simulink model "UUV_FD"  (R2018a)
settings: Solver=FixedStepAuto  StartTime=0.0  StopTime=25  FixedStep=0.01  RelTol=1e-3  EnableMultiTasking=on
settings Model: Creator=Alireza  LastModifiedBy=7385281
settings DataIOCC: LimitDataPoints=on  SaveFormat=Array  SignalLoggingSaveFormat=ModelDataLogs
settings OptimizationCC: ExpressionDepthLimit=2147483647  LifeSpan=inf
settings DebuggingCC: UnderspecifiedInitializationDetection=Classic  MergeDetectMultiDrivingBlocksExec=none  SolverPrmCheckMsg=warning  FcnCallInpInsideContextMsg=warning  AllowSymbolicDim=off  StateNameClashWarn=warning  SFUnexpectedBacktrackingDiag=warning  SFNoUnconditionalDefaultTransitionDiag=warning  SFExecutionAtInitializationDiag=none
settings HardwareCC: ProdBitPerPointer=32  ProdBitPerSizeT=32  ProdBitPerPtrDiffT=32  ProdLargestAtomicFloat=None  ProdIntDivRoundTo=Undefined  ProdEndianess=Unspecified  ProdWordSize=32  ProdHWDeviceType=32-bit Generic
settings ModelReferenceCC: PropagateSignalLabelsOutOfModel=off
settings CodeAppCC: StateflowObjectComments=on
settings GRTTargetCC: TargetLangStandard=C89/C90 (ANSI)  GeneratePreprocessorConditionals=Disable all  CombineOutputUpdateFcns=off  GRTInterface=on
settings ConfigComp: CovMetricSettings=dw  CovHtmlReporting=on  CovSaveCumulativeToWorkspaceVar=on  CovSaveSingleToWorkspaceVar=on  CovExternalEMLEnable=off

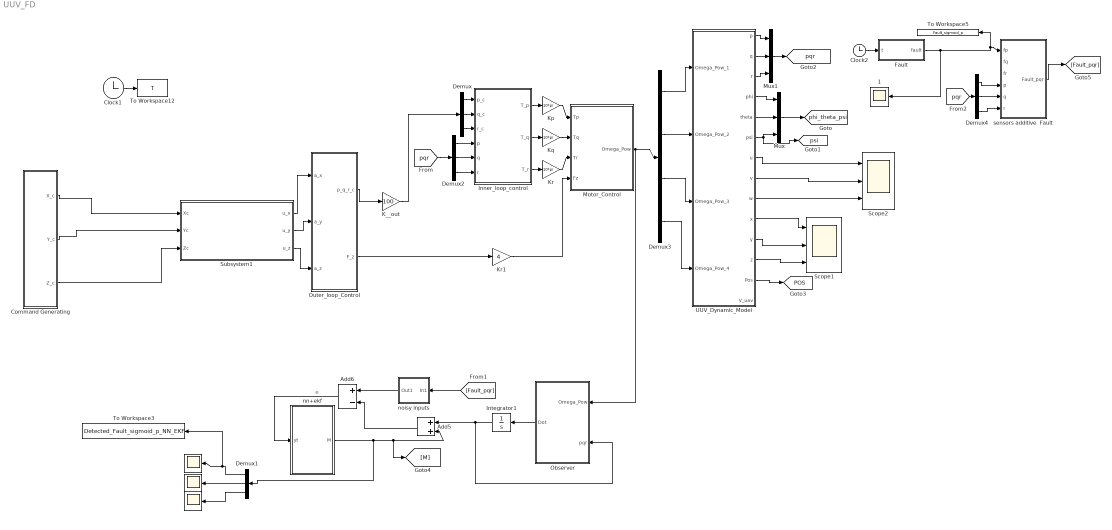
== system UUV_FD ==
  note: e
  "     " : Scope
  "      " : Scope
  "          " : Scope
  "     1" : Scope
  Add5 : Sum
  Add6 : Sum  Inputs=+-  OutDataTypeStr=Inherit: Same as accumulator
  Clock1 : Clock
  Clock2 : Clock
  Command Generating : Subsystem
  Demux{,1..2,4} (4 alike) : Demux  Outputs=3
  Demux3 : Demux
  Fault : MATLAB Function  TreatAsAtomicUnit=on
  Inner_loop_control : MATLAB Function  TreatAsAtomicUnit=on
  Integrator1 : Integrator  InitialCondition=[0.0001;0.0001;0.0001]
  K__out : Gain  Gain=100
  Kp : Gain  Gain=10*pi
  Kq : Gain  Gain=10*pi
  Kr : Gain  Gain=10*pi
  Kr1 : Gain  Gain=4
  Motor_Control : MATLAB Function  TreatAsAtomicUnit=on
  Mux : Mux  Inputs=3
  Mux1 : Mux  Inputs=3
  Observer : MATLAB Function  TreatAsAtomicUnit=on
  Outer_loop_Control : Subsystem
  Scope1 : Scope  NumInputPorts=3
  Scope2 : Scope  NumInputPorts=3
  Subsystem1 : Subsystem
  To Workspace12 : ToWorkspace  VariableName=T  SampleTime=-1
  To Workspace3 : ToWorkspace  VariableName=Detected_Fault_sigmoid_p_NN_EKF  SampleTime=-1
  To Workspace5 : ToWorkspace  VariableName=Fault_sigmoid_p  SampleTime=-1
  UUV_Dynamic_Model : Subsystem
  nn+ekf : Subsystem
  noisy inputs : Subsystem
  "sensors additive  Fault " : MATLAB Function  TreatAsAtomicUnit=on
  tag scope: POS=global, phi_theta_psi=global, pqr=global, psi=global
  wires:
  UUV_Dynamic_Model/4(phi) -> Mux/1
  UUV_Dynamic_Model/5(theta) -> Mux/2
  UUV_Dynamic_Model/6(psi) -> [psi], Mux/3
  Mux/1 -> [phi_theta_psi]
  Inner_loop_control/1(T_p) -> Kp/1
  Inner_loop_control/2(T_q) -> Kq/1
  Inner_loop_control/3(T_r) -> Kr/1
  UUV_Dynamic_Model/1(p) -> Mux1/1
  UUV_Dynamic_Model/2(q) -> Mux1/2
  UUV_Dynamic_Model/3(r) -> Mux1/3
  Mux1/1 -> [pqr]
  Demux2/1 -> Inner_loop_control/4(p)
  Demux2/2 -> Inner_loop_control/5(q)
  Demux2/3 -> Inner_loop_control/6(r)
  [pqr] -> Demux2/1
  K__out/1 -> Demux/1
  Demux/1 -> Inner_loop_control/1(p_c)
  Demux/2 -> Inner_loop_control/2(q_c)
  Demux/3 -> Inner_loop_control/3(r_c)
  UUV_Dynamic_Model/10(x) -> Scope1/1
  UUV_Dynamic_Model/11(y) -> Scope1/2
  UUV_Dynamic_Model/12(z) -> Scope1/3
  UUV_Dynamic_Model/7(u) -> Scope2/1
  UUV_Dynamic_Model/8(v) -> Scope2/2
  UUV_Dynamic_Model/9(w) -> Scope2/3
  UUV_Dynamic_Model/13(Pos) -> [POS]
  Motor_Control/1(Omega_Pow) -> Demux3/1, Observer/1(Omega_Pow)
  Demux3/1 -> UUV_Dynamic_Model/1(Omega_Pow_1)
  Demux3/3 -> UUV_Dynamic_Model/3(Omega_Pow_3)
  Demux3/4 -> UUV_Dynamic_Model/4(Omega_Pow_4)
  Kp/1 -> Motor_Control/1(Tp)
  Kq/1 -> Motor_Control/2(Tq)
  Kr/1 -> Motor_Control/3(Tr)
  Demux3/2 -> UUV_Dynamic_Model/2(Omega_Pow_2)
  Command Generating/1(X_c) -> Subsystem1/1(Xc)
  Command Generating/2(Y_c) -> Subsystem1/2(Yc)
  Command Generating/3(Z_c) -> Subsystem1/3(Zc)
  Clock1/1 -> To Workspace12/1
  Subsystem1/1(u_x) -> Outer_loop_Control/1(a_x)
  Subsystem1/2(u_y) -> Outer_loop_Control/2(a_y)
  Subsystem1/3(u_z) -> Outer_loop_Control/3(a_z)
  Outer_loop_Control/1(p_q_r_c) -> K__out/1
  Outer_loop_Control/2(F_z) -> Kr1/1
  Kr1/1 -> Motor_Control/4(Fz)
  "sensors additive  Fault "/1(Fault_pqr) -> [Fault_pqr]
  Fault/1(fault) -> To Workspace5/1, "sensors additive  Fault "/1(fp), "     1"/1
  Observer/1(Dot) -> Integrator1/1
  Integrator1/1 -> Add5/1, Observer/2(pqr)
  Add5/1 -> Add6/2
  Add6/1 -> nn+ekf/1(yt)
  nn+ekf/1(M) -> Add5/2, [M], Demux1/1
  Demux1/3 -> "          "/1
  Demux1/1 -> "     "/1, To Workspace3/1
  Demux1/2 -> "      "/1
  [Fault_pqr] -> noisy inputs/1(In1)
  noisy inputs/1(Out1) -> Add6/1
  [pqr] -> Demux4/1
  Demux4/3 -> "sensors additive  Fault "/6(r)
  Demux4/2 -> "sensors additive  Fault "/5(q)
  Demux4/1 -> "sensors additive  Fault "/4(p)
  Clock2/1 -> Fault/1(t)

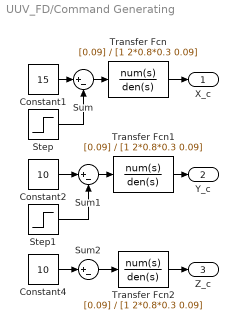
== system UUV_FD/Command Generating ==
  Constant1 : Constant  Value=15
  Constant2 : Constant  Value=10
  Constant4 : Constant  Value=10
  Step : Step  Time=30  After=15  SampleTime=0
  Step1 : Step  Time=15  After=10  SampleTime=0
  Sum : Sum  Inputs=|+-
  Sum1 : Sum  Inputs=|+-
  Sum2 : Sum  Inputs=|+-
  Transfer Fcn : TransferFcn  Numerator=[0.09]  Denominator=[1 2*0.8*0.3 0.09]
  Transfer Fcn1 : TransferFcn  Numerator=[0.09]  Denominator=[1 2*0.8*0.3 0.09]
  Transfer Fcn2 : TransferFcn  Numerator=[0.09]  Denominator=[1 2*0.8*0.3 0.09]
  X_c : Outport
  Y_c : Outport  Port=2
  Z_c : Outport  Port=3
  wires:
  Constant4/1 -> Sum2/1
  Transfer Fcn1/1 -> Y_c/1
  Transfer Fcn/1 -> X_c/1
  Constant2/1 -> Sum1/1
  Constant1/1 -> Sum/1
  Step/1 -> Sum/2
  Sum/1 -> Transfer Fcn/1
  Sum1/1 -> Transfer Fcn1/1
  Sum2/1 -> Transfer Fcn2/1
  Step1/1 -> Sum1/2
  Transfer Fcn2/1 -> Z_c/1

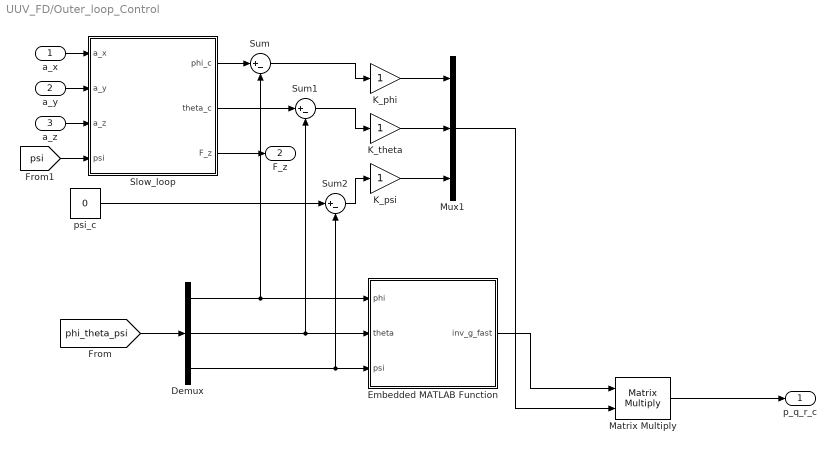
== system UUV_FD/Outer_loop_Control ==
  a_x : Inport
  a_y : Inport  Port=2
  a_z : Inport  Port=3
  Demux : Demux  Outputs=3
  Embedded MATLAB Function : MATLAB Function  TreatAsAtomicUnit=on
  K_phi : Gain
  K_psi : Gain
  K_theta : Gain
  Matrix Multiply : Product  Multiplication=Matrix(*)
  Mux1 : Mux  Inputs=3
  Slow_loop : MATLAB Function  TreatAsAtomicUnit=on
  Sum : Sum  Inputs=|+-
  Sum1 : Sum  Inputs=|+-
  Sum2 : Sum  Inputs=|+-
  psi_c : Constant  Value=0
  p_q_r_c : Outport
  F_z : Outport  Port=2
  wires:
  Sum1/1 -> K_theta/1
  Slow_loop/2(theta_c) -> Sum1/1
  Sum/1 -> K_phi/1
  Slow_loop/1(phi_c) -> Sum/1
  [phi_theta_psi] -> Demux/1
  Demux/1 -> Embedded MATLAB Function/1(phi), Sum/2
  Demux/2 -> Embedded MATLAB Function/2(theta), Sum1/2
  Demux/3 -> Embedded MATLAB Function/3(psi), Sum2/2
  psi_c/1 -> Sum2/1
  Sum2/1 -> K_psi/1
  [psi] -> Slow_loop/4(psi)
  K_phi/1 -> Mux1/1
  K_theta/1 -> Mux1/2
  K_psi/1 -> Mux1/3
  a_x/1 -> Slow_loop/1(a_x)
  a_y/1 -> Slow_loop/2(a_y)
  a_z/1 -> Slow_loop/3(a_z)
  Mux1/1 -> Matrix Multiply/2
  Slow_loop/3(F_z) -> F_z/1
  Embedded MATLAB Function/1(inv_g_fast) -> Matrix Multiply/1
  Matrix Multiply/1 -> p_q_r_c/1

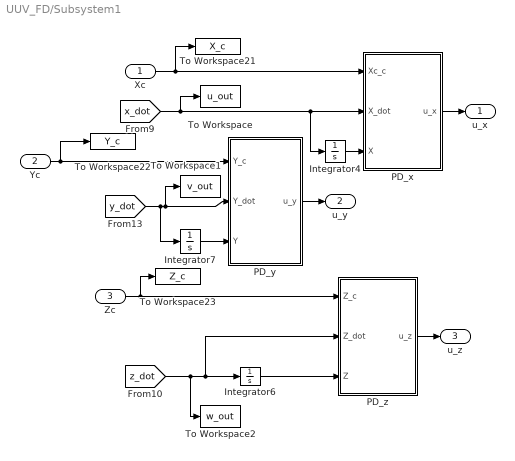
== system UUV_FD/Subsystem1 ==
  Xc : Inport
  Yc : Inport  Port=2
  Zc : Inport  Port=3
  Integrator4 : Integrator
  Integrator6 : Integrator
  Integrator7 : Integrator
  PD_x : Subsystem
  PD_y : Subsystem
  PD_z : Subsystem
  To Workspace : ToWorkspace  VariableName=u_out  SampleTime=-1
  To Workspace1 : ToWorkspace  VariableName=v_out  SampleTime=-1
  To Workspace2 : ToWorkspace  VariableName=w_out  SampleTime=-1
  To Workspace21 : ToWorkspace  VariableName=X_c  SampleTime=-1
  To Workspace22 : ToWorkspace  VariableName=Y_c  SampleTime=-1
  To Workspace23 : ToWorkspace  VariableName=Z_c  SampleTime=-1
  u_x : Outport
  u_y : Outport  Port=2
  u_z : Outport  Port=3
  wires:
  PD_z/1(u_z) -> u_z/1
  PD_y/1(u_y) -> u_y/1
  PD_x/1(u_x) -> u_x/1
  Zc/1 -> PD_z/1(Z_c), To Workspace23/1
  Yc/1 -> To Workspace22/1, PD_y/1(Y_c)
  Xc/1 -> PD_x/1(Xc_c), To Workspace21/1
  Integrator7/1 -> PD_y/3(Y)
  [x_dot] -> To Workspace/1, Integrator4/1, PD_x/2(X_dot)
  Integrator4/1 -> PD_x/3(X)
  [y_dot] -> PD_y/2(Y_dot), To Workspace1/1, Integrator7/1
  [z_dot] -> To Workspace2/1, Integrator6/1, PD_z/2(Z_dot)
  Integrator6/1 -> PD_z/3(Z)

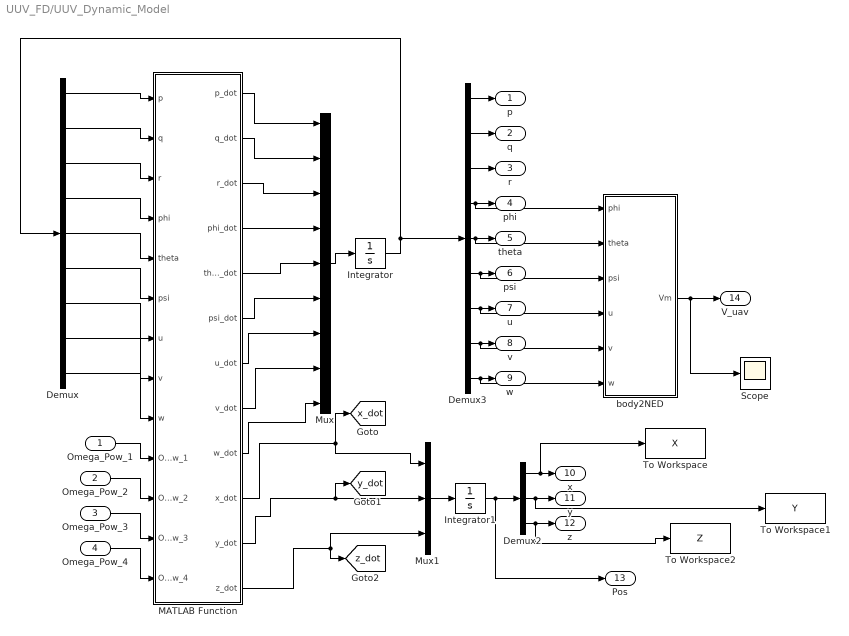
== system UUV_FD/UUV_Dynamic_Model ==
  Omega_Pow_1 : Inport
  Omega_Pow_2 : Inport  Port=2
  Omega_Pow_3 : Inport  Port=3
  Omega_Pow_4 : Inport  Port=4
  Demux : Demux  Outputs=9
  Demux2 : Demux  Outputs=3
  Demux3 : Demux  Outputs=9
  Integrator : Integrator  InitialCondition=[0.0001;0.0001;0.0001;0.00001;0.0001;0.0001;0.0001;0.0001;0.0001]
  Integrator1 : Integrator
  MATLAB Function : MATLAB Function  TreatAsAtomicUnit=on
  Mux : Mux  Inputs=9
  Mux1 : Mux  Inputs=3
  Scope : Scope
  To Workspace : ToWorkspace  VariableName=X  SampleTime=-1
  To Workspace1 : ToWorkspace  VariableName=Y  SampleTime=-1
  To Workspace2 : ToWorkspace  VariableName=Z  SampleTime=-1
  body2NED : MATLAB Function  TreatAsAtomicUnit=on
  p : Outport
  q : Outport  Port=2
  r : Outport  Port=3
  phi : Outport  Port=4
  theta : Outport  Port=5
  psi : Outport  Port=6
  u : Outport  Port=7
  v : Outport  Port=8
  w : Outport  Port=9
  x : Outport  Port=10
  y : Outport  Port=11
  z : Outport  Port=12
  Pos : Outport  Port=13
  V_uav : Outport  Port=14
  tag scope: x_dot=global, y_dot=global, z_dot=global
  wires:
  MATLAB Function/1(p_dot) -> Mux/1
  MATLAB Function/2(q_dot) -> Mux/2
  MATLAB Function/3(r_dot) -> Mux/3
  MATLAB Function/4(phi_dot) -> Mux/4
  MATLAB Function/5(theta_dot) -> Mux/5
  MATLAB Function/6(psi_dot) -> Mux/6
  MATLAB Function/7(u_dot) -> Mux/7
  MATLAB Function/8(v_dot) -> Mux/8
  MATLAB Function/9(w_dot) -> Mux/9
  Mux/1 -> Integrator/1
  Demux/1 -> MATLAB Function/1(p)
  Demux/2 -> MATLAB Function/2(q)
  Demux/3 -> MATLAB Function/3(r)
  Demux/4 -> MATLAB Function/4(phi)
  Demux/5 -> MATLAB Function/5(theta)
  Demux/6 -> MATLAB Function/6(psi)
  Demux/7 -> MATLAB Function/7(u)
  Demux/8 -> MATLAB Function/8(v)
  Demux/9 -> MATLAB Function/9(w)
  Integrator/1 -> Demux/1, Demux3/1
  MATLAB Function/10(x_dot) -> [x_dot], Mux1/1
  MATLAB Function/11(y_dot) -> Mux1/2, [y_dot]
  MATLAB Function/12(z_dot) -> [z_dot], Mux1/3
  Mux1/1 -> Integrator1/1
  Integrator1/1 -> Demux2/1, Pos/1
  Demux3/1 -> p/1
  Demux3/2 -> q/1
  Demux3/3 -> r/1
  Demux3/4 -> phi/1, body2NED/1(phi)
  Demux3/5 -> theta/1, body2NED/2(theta)
  Demux3/6 -> psi/1, body2NED/3(psi)
  Demux3/7 -> u/1, body2NED/4(u)
  Demux3/8 -> v/1, body2NED/5(v)
  Demux3/9 -> w/1, body2NED/6(w)
  Omega_Pow_1/1 -> MATLAB Function/10(Omega_Pow_1)
  Demux2/1 -> x/1, To Workspace/1
  Demux2/2 -> y/1, To Workspace1/1
  Omega_Pow_2/1 -> MATLAB Function/11(Omega_Pow_2)
  Demux2/3 -> z/1, To Workspace2/1
  Omega_Pow_3/1 -> MATLAB Function/12(Omega_Pow_3)
  Omega_Pow_4/1 -> MATLAB Function/13(Omega_Pow_4)
  body2NED/1(Vm) -> V_uav/1, Scope/1

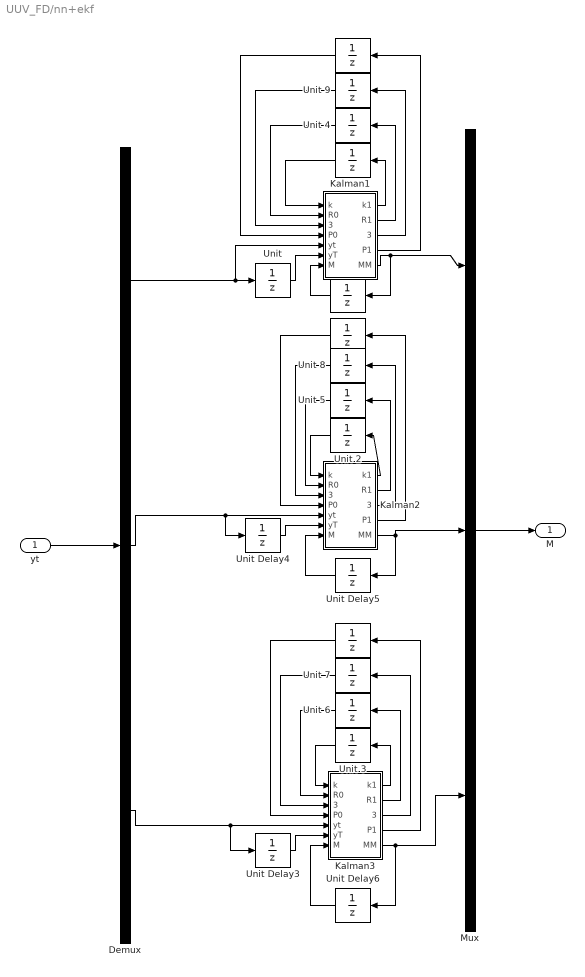
== system UUV_FD/nn+ekf ==
  yt : Inport
  " " : UnitDelay  InitialCondition=1  SampleTime=-1
  "  " : UnitDelay  InitialCondition=5*eye(3)  SampleTime=-1
  "   " : UnitDelay  InitialCondition=5*eye(3)  SampleTime=-1
  "      " : UnitDelay  InitialCondition=.01  SampleTime=-1
  "                " : UnitDelay  InitialCondition=10*eye(3)  SampleTime=-1
  Demux : Demux  Outputs=3
  Kalman1 : MATLAB Function  TreatAsAtomicUnit=on
  Kalman2 : MATLAB Function  TreatAsAtomicUnit=on
  Kalman3 : MATLAB Function  TreatAsAtomicUnit=on
  Mux : Mux  Inputs=3
  "Unit " : UnitDelay  SampleTime=-1
  Unit 2 : UnitDelay  InitialCondition=1  SampleTime=-1
  Unit 3 : UnitDelay  InitialCondition=1  SampleTime=-1
  Unit 4 : UnitDelay  InitialCondition=.00002  SampleTime=-1
  Unit 5 : UnitDelay  InitialCondition=.00002  SampleTime=-1
  Unit 6 : UnitDelay  InitialCondition=.00002  SampleTime=-1
  Unit 7 : UnitDelay  InitialCondition=[1;1;1]  SampleTime=-1
  Unit 8 : UnitDelay  InitialCondition=[1;.5;.5]  SampleTime=-1
  Unit 9 : UnitDelay  InitialCondition=[1;.5;.5]  SampleTime=-1
  Unit Delay3 : UnitDelay  SampleTime=-1
  Unit Delay4 : UnitDelay  SampleTime=-1
  Unit Delay5 : UnitDelay  InitialCondition=.01  SampleTime=-1
  Unit Delay6 : UnitDelay  InitialCondition=.01  SampleTime=-1
  M : Outport
  wires:
  "                "/1 -> Kalman3/4(P0)
  Kalman3/4(P1) -> "                "/1
  "   "/1 -> Kalman2/4(P0)
  Kalman2/4(P1) -> "   "/1
  Unit 8/1 -> Kalman2/3(teta0)
  Kalman2/3(teta1) -> Unit 8/1
  Unit 7/1 -> Kalman3/3(teta0)
  Kalman3/3(teta1) -> Unit 7/1
  Unit 6/1 -> Kalman3/2(R0)
  Kalman3/2(R1) -> Unit 6/1
  Unit 5/1 -> Kalman2/2(R0)
  Kalman2/2(R1) -> Unit 5/1
  Unit 3/1 -> Kalman3/1(k)
  Kalman3/1(k1) -> Unit 3/1
  Unit 2/1 -> Kalman2/1(k)
  Kalman2/1(k1) -> Unit 2/1
  Kalman3/5(MM) -> Unit Delay6/1, Mux/3
  Unit Delay5/1 -> Kalman2/7(M)
  Unit Delay4/1 -> Kalman2/6(yT)
  Unit Delay6/1 -> Kalman3/7(M)
  Unit Delay3/1 -> Kalman3/6(yT)
  Demux/2 -> Kalman2/5(yt), Unit Delay4/1
  Kalman2/5(MM) -> Unit Delay5/1, Mux/2
  Demux/3 -> Kalman3/5(yt), Unit Delay3/1
  Mux/1 -> M/1
  yt/1 -> Demux/1
  "  "/1 -> Kalman1/4(P0)
  Kalman1/4(P1) -> "  "/1
  Unit 9/1 -> Kalman1/3(teta0)
  Kalman1/3(teta1) -> Unit 9/1
  Unit 4/1 -> Kalman1/2(R0)
  Kalman1/2(R1) -> Unit 4/1
  " "/1 -> Kalman1/1(k)
  Kalman1/1(k1) -> " "/1
  "      "/1 -> Kalman1/7(M)
  "Unit "/1 -> Kalman1/6(yT)
  Demux/1 -> Kalman1/5(yt), "Unit "/1
  Kalman1/5(MM) -> "      "/1, Mux/1

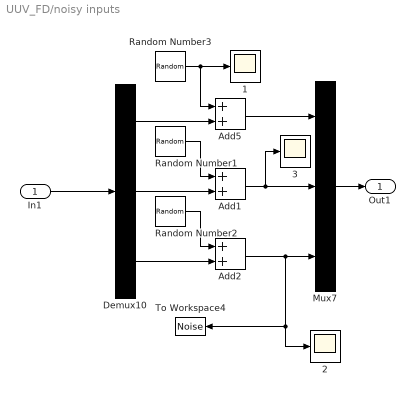
== system UUV_FD/noisy inputs ==
  In1 : Inport
  "     1" : Scope
  "     2" : Scope
  "     3" : Scope
  Add1 : Sum
  Add2 : Sum
  Add5 : Sum
  Demux10 : Demux  Outputs=3
  Mux7 : Mux  Inputs=3
  Random Number1 : RandomNumber  Variance=(1*pi/180)^2  Seed=18
  Random Number2 : RandomNumber  Variance=(1*pi/180)^2  Seed=40
  Random Number3 : RandomNumber  Variance=(1*pi/180)^2  Seed=68
  To Workspace4 : ToWorkspace  VariableName=Noise  SampleTime=-1
  Out1 : Outport
  wires:
  In1/1 -> Demux10/1
  Mux7/1 -> Out1/1
  Random Number3/1 -> Add5/1, "     1"/1
  Demux10/1 -> Add5/2
  Add5/1 -> Mux7/1
  Random Number1/1 -> Add1/1
  Demux10/2 -> Add1/2
  Add1/1 -> Mux7/2, "     3"/1
  Random Number2/1 -> Add2/1
  Demux10/3 -> Add2/2
  Add2/1 -> Mux7/3, "     2"/1, To Workspace4/1

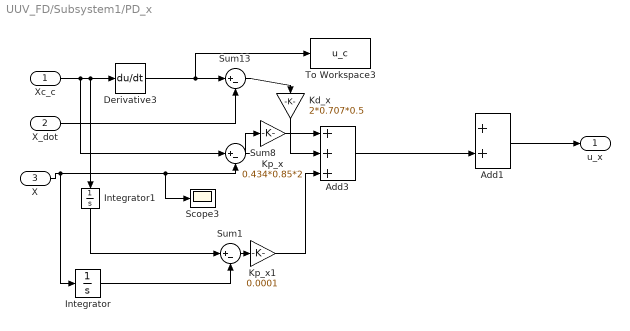
== system UUV_FD/Subsystem1/PD_x ==
  Xc_c : Inport
  X_dot : Inport  Port=2
  X : Inport  Port=3
  Add1 : Sum
  Add3 : Sum  Inputs=+++
  Derivative3 : Derivative
  Integrator : Integrator
  Integrator1 : Integrator
  Kd_x : Gain  Gain=2*0.707*0.5
  Kp_x : Gain  Gain=0.434*0.85*2
  Kp_x1 : Gain  Gain=0.0001
  Scope3 : Scope
  Sum1 : Sum  Inputs=|+-
  Sum13 : Sum  Inputs=|+-
  Sum8 : Sum  Inputs=|+-
  To Workspace3 : ToWorkspace  VariableName=u_c  SampleTime=-1
  u_x : Outport
  wires:
  Add3/1 -> Add1/2
  Add1/1 -> u_x/1
  Kp_x1/1 -> Add3/3
  Integrator1/1 -> Sum1/1
  Integrator/1 -> Sum1/2
  Sum1/1 -> Kp_x1/1
  X_dot/1 -> Sum13/2
  Xc_c/1 -> Integrator1/1, Derivative3/1, Sum8/1
  Kp_x/1 -> Add3/2
  Kd_x/1 -> Add3/1
  Sum13/1 -> Kd_x/1
  Derivative3/1 -> To Workspace3/1, Sum13/1
  X/1 -> Integrator/1, Sum8/2, Scope3/1
  Sum8/1 -> Kp_x/1

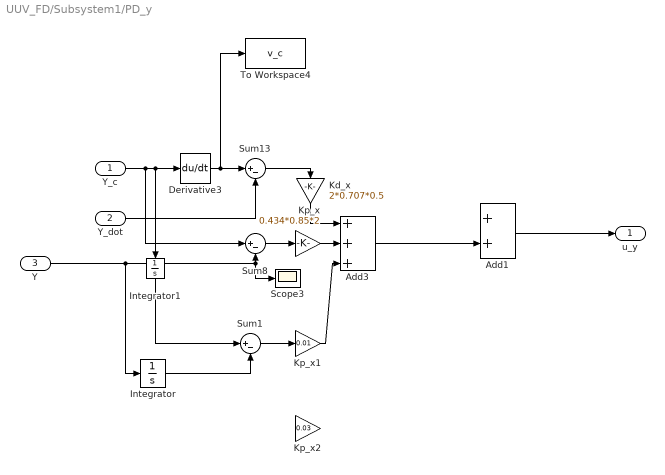
== system UUV_FD/Subsystem1/PD_y ==
  Y_c : Inport
  Y_dot : Inport  Port=2
  Y : Inport  Port=3
  Add1 : Sum
  Add3 : Sum  Inputs=+++
  Derivative3 : Derivative
  Integrator : Integrator
  Integrator1 : Integrator
  Kd_x : Gain  Gain=2*0.707*0.5
  Kp_x : Gain  Gain=0.434*0.85*2
  Kp_x1 : Gain  Gain=0.01
  Kp_x2 : Gain  Gain=0.03
  Scope3 : Scope
  Sum1 : Sum  Inputs=|+-
  Sum13 : Sum  Inputs=|+-
  Sum8 : Sum  Inputs=|+-
  To Workspace4 : ToWorkspace  VariableName=v_c  SampleTime=-1
  u_y : Outport
  wires:
  Add1/1 -> u_y/1
  Add3/1 -> Add1/2
  Y_dot/1 -> Sum13/2
  Y_c/1 -> Integrator1/1, Derivative3/1, Sum8/1
  Kp_x1/1 -> Add3/3
  Integrator1/1 -> Sum1/1
  Integrator/1 -> Sum1/2
  Sum1/1 -> Kp_x1/1
  Kp_x/1 -> Add3/2
  Kd_x/1 -> Add3/1
  Sum13/1 -> Kd_x/1
  Derivative3/1 -> Sum13/1, To Workspace4/1
  Y/1 -> Integrator/1, Sum8/2, Scope3/1
  Sum8/1 -> Kp_x/1

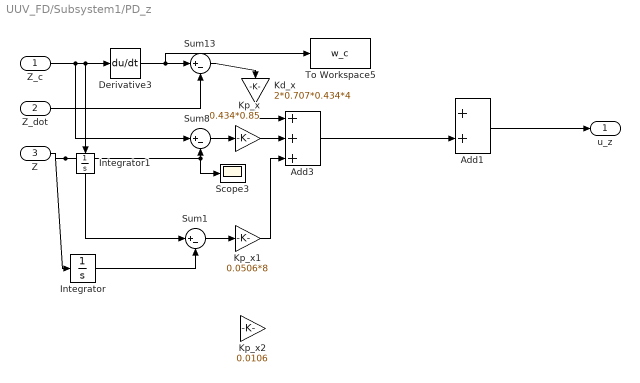
== system UUV_FD/Subsystem1/PD_z ==
  Z_c : Inport
  Z_dot : Inport  Port=2
  Z : Inport  Port=3
  Add1 : Sum
  Add3 : Sum  Inputs=+++
  Derivative3 : Derivative
  Integrator : Integrator
  Integrator1 : Integrator
  Kd_x : Gain  Gain=2*0.707*0.434*4
  Kp_x : Gain  Gain=0.434*0.85
  Kp_x1 : Gain  Gain=0.0506*8
  Kp_x2 : Gain  Gain=0.0106
  Scope3 : Scope
  Sum1 : Sum  Inputs=|+-
  Sum13 : Sum  Inputs=|+-
  Sum8 : Sum  Inputs=|+-
  To Workspace5 : ToWorkspace  VariableName=w_c  SampleTime=-1
  u_z : Outport
  wires:
  Add3/1 -> Add1/2
  Add1/1 -> u_z/1
  Z_dot/1 -> Sum13/2
  Z_c/1 -> Integrator1/1, Derivative3/1, Sum8/1
  Kp_x1/1 -> Add3/3
  Integrator1/1 -> Sum1/1
  Integrator/1 -> Sum1/2
  Sum1/1 -> Kp_x1/1
  Kp_x/1 -> Add3/2
  Kd_x/1 -> Add3/1
  Sum13/1 -> Kd_x/1
  Derivative3/1 -> To Workspace5/1, Sum13/1
  Z/1 -> Integrator/1, Sum8/2, Scope3/1
  Sum8/1 -> Kp_x/1

== matlab function UUV_FD/Outer_loop_Control/Embedded MATLAB Function ==
  data: phi input; inv_g_fast output; theta input; psi input
function inv_g_fast = fcn(phi,theta,psi)
g=[1 sin(phi)*tan(theta) cos(phi)*tan(theta)
    0 cos(phi) -sin(phi)
    0 sin(phi)/cos(theta) cos(phi)/cos(theta)];
inv_g_fast=inv(g);

== matlab function UUV_FD/UUV_Dynamic_Model/MATLAB Function ==
  data: p input; q input; r input; phi input; theta input; psi input; u input; p_dot output; v input; w input; Omega_Pow_1 input; Omega_Pow_2 input; Omega_Pow_3 input; Omega_Pow_4 input; q_dot output; r_dot output; phi_dot output; theta_dot output; psi_dot output; u_dot output; v_dot output; w_dot output; x_dot output; y_dot output; z_dot output
function [p_dot,q_dot,r_dot,phi_dot,theta_dot,psi_dot,u_dot,v_dot,w_dot,x_dot,y_dot,z_dot] = fcn(p,q,r,phi,theta,psi,u,v,w,Omega_Pow_1,Omega_Pow_2,Omega_Pow_3,Omega_Pow_4)
% Assumumptions
    % Relative low speed, lift forces neglected
    % AUV sysmetric about xz, yz, xy plane
        % can decouple dof
        % Coriolis Matrices are ignored
    % aligning moment ensures stability
    % no trhust in the surge and sway directions
    % B frame is at center of gravity
    % No enviromental disturbances such as current or wind
    % Thrust is generated at the same plane as the center of gravity
    % Added mass parameters are estimated 50% of rigid body mass. Typically
        % between 10% and 100% of rigid body mass parameters
%%%%%%%%%%%%%%%%%%%%%%%%%%%%%%%%%%%%%%%%%%%%%%%%%%%%%%%%%%%%%%%%%%%%%%%%%%
% INPUTS
% p - roll rate
% q - pitch rate
% r - yaw rate
% phi - roll
% theta - pitch
% psi - yaw
% u - surge rate
% v - sway rate
% w - heave rate
% Omega_1,2,3,4 - angular velocities of vertical thrusters
%%%%%%%%%%%%%%%%%%%%%%%%%%%%%%%%%%%%%%%%%%%%%%%%%%%%%%%%%%%%%%%%%%%%%%%%%%%
% UUV Constant Parameters (Kambara)
mass = 175; %[kg]    mass
Ixx = 14;   %[kg m^2]   moment of area about x
Iyy = 13;   %[kg m^2]   moment of area about y
Izz = 16;   %[kg m^2]   moment of area about z
Xdu = mass*0.5;   %added mass term   
Ydv = mass*0.5;   %added mass term
Zdw = mass*0.5;   %added mass term
Kdp = Ixx*0.5;    %added mass term
Mdq = Iyy*0.5;    %added mass term
Ndr = Izz*0.5;    %added mass term
Xuu = 90;   %[Ns^2/m^2] quadratic drag term in u
Yvv = 90;   %[Ns^2/m^2] quadratic drag term in v
Zww = 120;  %[Ns^2/m^2] quadratic drag term in w
Kpp = 0;    %[Ns^2/m^2] quadratic drag term in p
Mqq = 0;    %[Ns^2/m^2] quadratic drag term in q
Nrr = 15;   %[Ns^2/m^2] quadratic drag term in r
xg = 0;     % Center of gravity, x
xb = 0;     % Center of buoyancy, x
yg = 0;     % Center of gravity, y
yb = 0;     % Center of buoyancy, y
zg = 0;     % Center of gravity, z
zb = 100;   % Center of buoyancy, z
Xu = 120;   % [Ns/m]   Linear Drag
Yv = 90;    % [Ns/m]   Linear Drag    
Zw = 150;   % [Ns/m]   Linear Drag
Kp = 0;     % [Ns/m]   Linear Drag
Mq = 0;     % [Ns/m]   Linear Drag
Nr = 18;    % [Ns/m]   Linear Drag 
L = 0.4;    % [m]   distance of thruster to center of gravity
K_f = 0.396;    % thrust coeffecient of thrusters
K_t = 0.338;    % Torque coeffeceint of thrusters
% Calculated Parameters/Enviorment
W = mass*9.81;  % [N] - weight
dens = 997; %[kg/m^3] - density
V = 151; %[L] - volume
V = V*0.001;    %Convert to m^3
B = dens*9.81*V;    %Buoyancy
Cd = 0.5;   %drag coeffeceint estimate
Af = .2921^2*pi()/4; %cross Section area

%%%%%%%%%%%%%%%%%%%%%%%%%%%%%%%%%%%%%%%%%%%%%%%%%%%%%%%%%%%%%%%%%%%%%%%%%%
% Calculates the force and moments from the thrusters 
% Moment about p
Tp=L*K_f*(Omega_Pow_1^2-Omega_Pow_2^2+Omega_Pow_3^2-Omega_Pow_4^2);

% Moment about q
Tq=L*K_f*(Omega_Pow_1^2+Omega_Pow_2^2-Omega_Pow_3^2-Omega_Pow_4^2);

% Moment about r
Tr=L*K_t*(Omega_Pow_1^2+Omega_Pow_2^2-Omega_Pow_3^2-Omega_Pow_4^2);

% Force in z direction
Fz=K_f*(Omega_Pow_1^2+Omega_Pow_2^2+Omega_Pow_3^2+Omega_Pow_4^2);

% mass matrices
    % Rigid Body Mass Matrix
mass_rb = [mass 0 0 0 0 0;...
            0 mass 0 0 0 0;...
            0 0 mass 0 0 0;...
            0 0 0 Ixx 0 0;...
            0 0 0 0 Iyy 0;...
            0 0 0 0 0 Izz];
        
     % Added Mass Matrix
mass_A = [Xdu 0 0 0 0 0;...
            0 Ydv 0 0 0 0;...
            0 0 Zdw 0 0 0;...
            0 0 0 Kdp 0 0;...
            0 0 0 0 Mdq 0;...
            0 0 0 0 0 Ndr];
        
imass = mass_rb + mass_A;

% Damping Matrices
    % Linear Damping Matrix
linear_damping = [Xu 0 0 0 0 0;...
                  0 Yv 0 0 0 0;...
                  0 0 Zw 0 0 0;...
                  0 0 0 Kp 0 0;...
                  0 0 0 0 Mq 0;...
                  0 0 0 0 0 Nr];
              
    % Quadratic Damping Matrix
quad_damping = [Xuu*abs(u) 0 0 0 0 0;...
                0 Yvv*abs(v) 0 0 0 0;...
                0 0 Zww*abs(w) 0 0 0;...
                0 0 0  Kpp*abs(p) 0 0;...
                0 0 0 0 Mqq*abs(q) 0;...
                0 0 0 0 0 Nrr*abs(r)];
            
damping = linear_damping + quad_damping;

%buoyancy matrix
buoy = [(W-B)*sin(theta);...
        -(W-B)*cos(theta)*sin(phi);...
        -(W-B)*cos(theta)*sin(phi);...
        -(yg*W-yb*B)*cos(theta)*cos(phi)+(zg*W-zb*B)*cos(theta)*cos(phi);...
        (zg*W-zb*B)*sin(theta)-(xg*W-xb*B)*cos(theta)*cos(phi);...
        -(xg*W-xb*B)*cos(theta)*sin(phi)-(yg*W-yb*B)*sin(theta)];
   
% Kinetic equations of motion, from Fossen, page 27. Eq 2.41-2.47 updated
% UUV
x_dot = u*cos(psi)*cos(theta) + v*(cos(psi)*sin(theta)*sin(phi)-sin(psi)*cos(phi)) + w*(sin(psi)*sin(phi)+cos(psi)*cos(phi)*sin(theta));
y_dot = u*sin(psi)*cos(theta) + v*(cos(psi)*cos(phi)+sin(phi)*sin(theta)*sin(psi)) + w*(sin(theta)*sin(psi)*cos(phi)-cos(psi)*sin(phi));
z_dot = -u*sin(theta) + v*cos(theta)*sin(phi) + w*cos(theta)*cos(phi);
phi_dot= p + q*sin(phi)*tan(theta) + r*cos(phi)*tan(theta);
theta_dot = q*cos(phi) - r*sin(phi);
psi_dot = q*sin(phi)/cos(theta) + r*cos(phi)/cos(theta);

% Kinematic Equations of motion % Updated for UUV
% Not including 2 horizantal thrusters
u_dot = -u*damping(1,1)/imass(1,1) - buoy(1,1)/imass(1,1);
v_dot = -v*damping(2,2)/imass(2,2) - buoy(2,1)/imass(2,2);
w_dot = -w*damping(3,3)/imass(3,3) - buoy(3,1)/imass(3,3)+Fz/imass(3,3);
p_dot = -p*damping(4,4)/imass(4,4) - buoy(4,1)/imass(4,4)+Tp/imass(4,4);
q_dot = -q*damping(5,5)/imass(5,5) - buoy(5,1)/imass(5,5)+Tq/imass(5,5);
r_dot = -r*damping(6,6)/imass(6,6) - buoy(6,1)/imass(6,6)+Tr/imass(6,6);

== matlab function UUV_FD/Outer_loop_Control/Slow_loop ==
  data: phi_c output; theta_c output; a_x input; a_y input; a_z input; F_z output; psi input
function [phi_c,theta_c,F_z] = fcn(a_x,a_y,a_z,psi)
g=9.81;
m=175; %kg (mass of quadrotor)
F_z=(a_z+g)*m;
phi_c=(a_x*sin(psi)-a_y*cos(psi))*m/F_z;
theta_c=(a_x*cos(psi)+a_y*sin(psi))*m/F_z;

== matlab function UUV_FD/Inner_loop_control ==
  data: p_c input; T_p output; q_c input; T_q output; T_r output; r_c input; p input; q input; r input
function [T_p,T_q,T_r] = fcn(p_c,q_c,r_c,p,q,r)
Ix=14; % kgm^2 Body of inertia of x axsis uuv
Iy=13;%kgm^2 Body of inertia of y axsis uuv
Iz=16;%kgm^2 Body of inertia of z axsis uuv

% Not updated yet
T_p=(p_c-p)*Ix;
T_q=(q_c-q)*Iy;
T_r=(r_c-r)*Iz;

== matlab function UUV_FD/Motor_Control ==
  data: Tp input; Omega_Pow output; Tq input; Tr input; Fz input
function Omega_Pow = fcn(Tp,Tq,Tr,Fz)
Kf=0.396; %N/(rad/s)^2 Force of UUV coefficient
Kt=0.338; %N/(rad/s)^2 Torque of UUV coefficient
L=0.4; %m Lever arm of vertical thrusters to center of gravity of UUV

% Lifting Force + Moments Coeffeccients
A = [Kf*L -Kf*L Kf*L -Kf*L;...
     Kf*L Kf*L -Kf*L -Kf*L;...
     Kt -Kt -Kt Kt;...
     Kf Kf Kf Kf];
 % Moments and lifting Force
 B = [Tp Tq Tr Fz]';
 
 % Calculates the angular velocity of the vertical thrusters.
 Omega_Pow_2 = A^(-1)*B;
Omega_Pow = sqrt(abs(Omega_Pow_2));

== matlab function UUV_FD/Fault ==
  data: t input; fault output
function fault = fcn(t)
t0=5;
omega=0.01;
if t<=t0
    fault=0;
else
    fault=1-exp(-omega*(t-t0));
end

== matlab function UUV_FD/Observer ==
  data: Omega_Pow input; Dot output; pqr input
function Dot   = fcn(Omega_Pow,pqr)
p=pqr(1);
q=pqr(2);
r=pqr(3);
Omega_Pow_1=Omega_Pow(1);
Omega_Pow_2=Omega_Pow(2);
Omega_Pow_3=Omega_Pow(3);
Omega_Pow_4=Omega_Pow(4);

% UUV Constant Parameters (Kambara)
mass = 175; %[kg]    mass
Ixx = 14;   %[kg m^2]   moment of area about x
Iyy = 13;   %[kg m^2]   moment of area about y
Izz = 16;   %[kg m^2]   moment of area about z
Xdu = mass*0.5;   %added mass term   
Ydv = mass*0.5;   %added mass term
Zdw = mass*0.5;   %added mass term
Kdp = Ixx*0.5;    %added mass term
Mdq = Iyy*0.5;    %added mass term
Ndr = Izz*0.5;    %added mass term
Xuu = 90;   %[Ns^2/m^2] quadratic drag term in u
Yvv = 90;   %[Ns^2/m^2] quadratic drag term in v
Zww = 120;  %[Ns^2/m^2] quadratic drag term in w
Kpp = 0;    %[Ns^2/m^2] quadratic drag term in p
Mqq = 0;    %[Ns^2/m^2] quadratic drag term in q
Nrr = 15;   %[Ns^2/m^2] quadratic drag term in r
xg = 0;     % Center of gravity, x
xb = 0;     % Center of buoyancy, x
yg = 0;     % Center of gravity, y
yb = 0;     % Center of buoyancy, y
zg = 0;     % Center of gravity, z
zb = 100;   % Center of buoyancy, z
Xu = 120;   % [Ns/m]   Linear Drag
Yv = 90;    % [Ns/m]   Linear Drag    
Zw = 150;   % [Ns/m]   Linear Drag
Kp = 0;     % [Ns/m]   Linear Drag
Mq = 0;     % [Ns/m]   Linear Drag
Nr = 18;    % [Ns/m]   Linear Drag 
K_f = 0.396;    % thrust coeffecient of thrusters
K_t = 0.338;    % Torque coeffeceint of thrusters
L = 0.4;    % [m]
% Calculated Parameters/Enviorment
W = mass*9.81;  % [N] - weight
dens = 997; %[kg/m^3] - density
V = 151; %[L] - volume
V = V*0.001;    %Convert to m^3
B = dens*9.81*V;    %Buoyancy
Cd = 0.5;   %drag coeffeceint estimate
Af = .2921^2*pi()/4; %cross Section area
u = 0;
v = 0;
w = 0;
theta=0;
phi=0;
psi=0;

%%%%%%%%%%%%%%%%%%%%%%%%%%%%%%%%%%%%%%%%%%%%%%%%%%%%%%%%%%%%%%%%%%%%%%%%%%
% Calculates the force and moments from the thrusters 
% Moment about p
Tp=L*K_f*(Omega_Pow_1^2-Omega_Pow_2^2+Omega_Pow_3^2-Omega_Pow_4^2);

% Moment about q
Tq=L*K_f*(Omega_Pow_1^2+Omega_Pow_2^2-Omega_Pow_3^2-Omega_Pow_4^2);

% Moment about r
Tr=L*K_t*(Omega_Pow_1^2+Omega_Pow_2^2-Omega_Pow_3^2-Omega_Pow_4^2);


% mass matrices
    % Rigid Body Mass Matrix
mass_rb = [mass 0 0 0 0 0;...
            0 mass 0 0 0 0;...
            0 0 mass 0 0 0;...
            0 0 0 Ixx 0 0;...
            0 0 0 0 Iyy 0;...
            0 0 0 0 0 Izz];
        
     % Added Mass Matrix
mass_A = [Xdu 0 0 0 0 0;...
            0 Ydv 0 0 0 0;...
            0 0 Zdw 0 0 0;...
            0 0 0 Kdp 0 0;...
            0 0 0 0 Mdq 0;...
            0 0 0 0 0 Ndr];
        
imass = mass_rb + mass_A;

% Damping Matrices
    % Linear Damping Matrix
linear_damping = [Xu 0 0 0 0 0;...
                  0 Yv 0 0 0 0;...
                  0 0 Zw 0 0 0;...
                  0 0 0 Kp 0 0;...
                  0 0 0 0 Mq 0;...
                  0 0 0 0 0 Nr];
              
    % Quadratic Damping Matrix
quad_damping = [Xuu*abs(u) 0 0 0 0 0;...
                0 Yvv*abs(v) 0 0 0 0;...
                0 0 Zww*abs(w) 0 0 0;...
                0 0 0  Kpp*abs(p) 0 0;...
                0 0 0 0 Mqq*abs(q) 0;...
                0 0 0 0 0 Nrr*abs(r)];
            
damping = linear_damping + quad_damping;

%buoyancy matrix
buoy = [(W-B)*sin(theta);...
        -(W-B)*cos(theta)*sin(phi);...
        -(W-B)*cos(theta)*sin(phi);...
        -(yg*W-yb*B)*cos(theta)*cos(phi)+(zg*W-zb*B)*cos(theta)*cos(phi);...
        (zg*W-zb*B)*sin(theta)-(xg*W-xb*B)*cos(theta)*cos(phi);...
        -(xg*W-xb*B)*cos(theta)*sin(phi)-(yg*W-yb*B)*sin(theta)];
%==============================

p_dot = -p*damping(4,4)/imass(4,4) - buoy(4,1)/imass(4,4)+Tp/imass(4,4);
q_dot = -q*damping(5,5)/imass(5,5) - buoy(5,1)/imass(5,5)+Tq/imass(5,5);
r_dot = -r*damping(6,6)/imass(6,6) - buoy(6,1)/imass(6,6)+Tr/imass(6,6);

Dot=[p_dot;q_dot;r_dot];

== matlab function UUV_FD/nn+ekf/Kalman1 ==
  data: k1 output; R1 output; teta1 output; P1 output; k input; R0 input; teta0 input; P0 input; MM output; yt input; yT input; M input
function [k1,R1,teta1,P1,MM]  = fcn(k,R0,teta0,P0,yt,yT,M)
eta=1.5;    % Change to improve based on model 0-3
Z=teta0(2)*M+teta0(3)*yT;
sigma=(1-exp(-Z))/(1+exp(-Z));
H=[sigma;teta0(1)*M*0.5*(1-sigma^2);teta0(1)*yT*0.5*(1-sigma^2)];
R1=R0+(yt^2-R0)/k;
K=P0*H*(((H'*P0*H)+R1)^(-1));
teta1=teta0+eta*K*(yt);
n=teta1(2)*M+teta1(3)*yT;
MM=teta1(1)*((1-exp(-n))/(1+exp(-n)));
P1=P0-K*H'*P0;
k1=k+1;

== matlab function UUV_FD/nn+ekf/Kalman2 ==
  data: k1 output; R1 output; teta1 output; P1 output; k input; R0 input; teta0 input; P0 input; MM output; yt input; yT input; M input
function [k1,R1,teta1,P1,MM]  = fcn(k,R0,teta0,P0,yt,yT,M)
eta=1;  % Change to improve based on model 0-3
Z=teta0(2)*M+teta0(3)*yT;
sigma=(1-exp(-Z))/(1+exp(-Z));
H=[sigma;teta0(1)*M*.5*(1-sigma^2);teta0(1)*yT*0.5*(1-sigma^2)];
R1=R0+(yt^2-R0)/k;
K=P0*H*(((H'*P0*H)+R1)^(-1));
teta1=teta0+eta*K*(yt);
n=teta1(2)*M+teta1(3)*yT;
MM=teta1(1)*((1-exp(-n))/(1+exp(-n)));
P1=P0-K*H'*P0;
k1=k+1;

== matlab function UUV_FD/nn+ekf/Kalman3 ==
  data: k1 output; R1 output; teta1 output; P1 output; k input; R0 input; teta0 input; P0 input; MM output; yt input; yT input; M input
function [k1,R1,teta1,P1,MM] = fcn(k,R0,teta0,P0,yt,yT,M)
eta=1;      % Change to improve based on model 0-3
Z=teta0(2)*M+teta0(3)*yT;
sigma=(1-exp(-Z))/(1+exp(-Z));
H=[sigma;teta0(1)*M*0.5*(1-sigma^2);teta0(1)*yT*0.5*(1-sigma^2)];
R1=R0+(yt^2-R0)/k;
K=P0*H*(((H'*P0*H)+R1)^(-1));
teta1=teta0+eta*K*(yt);
n=teta1(2)*M+teta1(3)*yT;
MM=teta1(1)*((1-exp(-n))/(1+exp(-n)));
P1=P0-K*H'*P0;
k1=k+1;

== matlab function UUV_FD/UUV_Dynamic_Model/body2NED ==
  data: phi input; theta input; psi input; u input; v input; w input; Vm output
function Vm= fcn(phi,theta,psi,u,v,w)
N=[cos(theta)*cos(psi) (sin(phi)*sin(theta)*cos(psi)-cos(phi)*sin(psi)) (cos(phi)*sin(theta)*cos(psi)+sin(phi)*sin(psi));
   -cos(theta)*sin(psi) -(sin(phi)*sin(theta)*sin(psi)+cos(phi)*cos(psi)) -(cos(phi)*sin(theta)*sin(psi) - sin(phi)*cos(psi));
   sin(theta) -sin(phi)*cos(theta) -cos(phi)*cos(theta)];
Vm=N*[u;v;w];
end

== matlab function UUV_FD/sensors additive  Fault  ==
  data: fp input; Fault_pqr output; fq input; fr input; p input; q input; r input
function Fault_pqr = fcn(fp,fq,fr,p,q,r)

Fault_pqr = [p;q;r]+[fp;fq;fr]+[.00060;.000001;.000001];
